simulink model "ovap_sim"  (R2025a)
settings: Solver=FixedStepAuto  StartTime=0.0  StopTime=100  FixedStep=0.002  RelTol=1e-3
undefined symbols (not defined in the file): X, Y, Z
libraries: sm_lib x88, nesl_utility x45, simulink_extras x31, slpidlib x8
(part 5 of 5)

== matlab function ovap_sim/2_Flight_Control_System/WPIN - 2/WPIN ==
  data: tau_des input; math_alpha input; math_beta input; r_mat input; math_thrust output; cmd_math_alpha output; cmd_math_beta output; h_eff input; kq input; coax_eff input; coax_tq_eff input; dir_top input; max_thrust input; W_weights input; F1 output; M1 output; F2 output; M2 output; F3 output; M3 output; F4 output; M4 output
function [math_thrust, cmd_math_alpha, cmd_math_beta, F1, M1, F2, M2, F3, M3, F4, M4] = WPIN_Core(tau_des, math_alpha, math_beta, ...
    r_mat, h_eff, kq, coax_eff, coax_tq_eff, dir_top, max_thrust, W_weights)
% KHỐI TOÁN HỌC THUẦN TÚY (KHÔNG CHỨA LOGIC PHẦN CỨNG)

    math_thrust = zeros(8,1); cmd_math_alpha = zeros(4,1); cmd_math_beta = zeros(4,1);
    
    F1 = zeros(3,1); M1 = zeros(3,1);
    F2 = zeros(3,1); M2 = zeros(3,1);
    F3 = zeros(3,1); M3 = zeros(3,1);
    F4 = zeros(3,1); M4 = zeros(3,1);
    
    tau_des = tau_des(:); math_alpha = math_alpha(:); math_beta = math_beta(:);

    % 1. Xây dựng ma trận Jacobian A (6x16)
    A = zeros(6, 16);
    for i = 1:4
        alpha = math_alpha(i); 
        beta = math_beta(i);
        
        R_s = [ cos(alpha),  sin(alpha)*sin(beta),  sin(alpha)*cos(beta);
                         0,            cos(beta),           -sin(beta);
               -sin(alpha),  cos(alpha)*sin(beta),  cos(alpha)*cos(beta)];
        
        r_pivot = r_mat(i,:)';
        r_prop_offset = R_s * [0; 0; -h_eff]; 
        r_total = r_pivot + r_prop_offset; 
        
        v_dir_neg = R_s * [0; 0; 1];
        
        idx = (i-1)*4;
        A(1:3, idx+1 : idx+3) = eye(3);
        A(4:6, idx+1 : idx+3) = [0 -r_total(3) r_total(2); r_total(3) 0 -r_total(1); -r_total(2) r_total(1) 0];
        A(4:6, idx+4)         = v_dir_neg; 
    end

    % 2. Ma trận Trọng số W 
    W_inv = diag([1./W_weights(1:3); 1./W_weights(4); 1./W_weights(1:3); 1./W_weights(4); ...
                  1./W_weights(1:3); 1./W_weights(4); 1./W_weights(1:3); 1./W_weights(4)]);

    % 3. Giải Giả nghịch đảo WPIN
    A_dagger = (W_inv * A') / (A * W_inv * A' + 1e-6 * eye(6));
    u_total = A_dagger * tau_des;

    % 4. Inverse Kinematics & Phân rã Đồng trục
    eta_c  = coax_eff;        
    lam_c  = coax_tq_eff; 
    c_q    = kq;
    
    for i = 1:4
        idx = (i-1)*4;
        Fi      = u_total(idx+1 : idx+3);
        M_delta = u_total(idx+4); 
        
        T_i = norm(Fi);
        if T_i > 0.01
            cmd_math_alpha(i) = atan2(-Fi(1), -Fi(3));
            cmd_math_beta(i)  = atan2(Fi(2), sqrt(Fi(1)^2 + Fi(3)^2));
        end
        
        F_local = [0; 0; -T_i];
        M_local = [0; 0; -M_delta];
        
        if i == 1
            F1 = F_local; M1 = M_local;
        elseif i == 2
            F2 = F_local; M2 = M_local;
        elseif i == 3
            F3 = F_local; M3 = M_local;
        elseif i == 4
            F4 = F_local; M4 = M_local;
        end
        
        delta_T = M_delta / (dir_top(i) * c_q);
        
        T_bot = (T_i - delta_T) / (eta_c + lam_c); 
        T_top = T_i - eta_c * T_bot;
        
        if T_bot < 0
            T_bot = 0;
            T_top = T_i; 
        end
        if T_top < 0
            T_top = 0;
            T_bot = T_i / eta_c; 
        end
        
        % Lưu mảng thrust nội bộ (Arm 1 -> Arm 4)
        math_thrust((i-1)*2 + 1) = min(T_top, max_thrust(2)); % Top
        math_thrust((i-1)*2 + 2) = min(T_bot, max_thrust(2)); % Bot
    end
end
